simulink model "opv_HDL_Coder_input"  (R2023a)
settings: Solver=VariableStepAuto  StartTime=0.0  StopTime=4*(1/sample_rate)  RelTol=1e-3
values from neighbouring files (symbols this model uses):
  sample_rate = samples_per_symbol*symbol_rate    (= 271000)    [opv.m]
libraries: hdlsllib x2, dspsigops x1
settings Model: Creator=matt  LastModifiedBy=matt

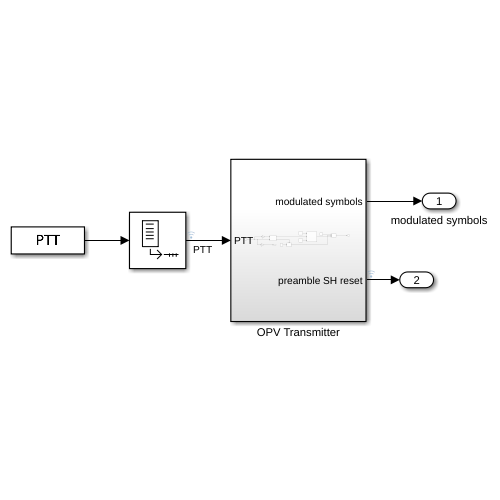
[thumbnail: Simulink's stored preview of the top-level diagram]
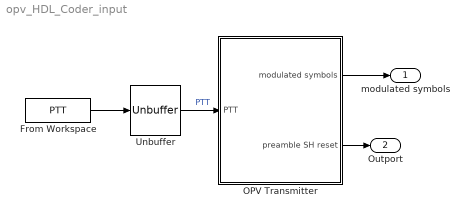
== system opv_HDL_Coder_input ==
  From Workspace : FromWorkspace  VariableName=PTT  OutDataTypeStr=boolean  SampleTime=1/sample_rate
  OPV Transmitter : Subsystem
      settings: LibrarySourceBlock=|
      | hdlsllib/Ports &
      | Subsystems/Subsystem
  Unbuffer : Unbuffer
  modulated symbols : Outport
  Outport : Outport  Port=2
  wires:
  From Workspace/1 -> Unbuffer/1
  Unbuffer/1 -> OPV Transmitter/1(PTT)  "PTT"
  OPV Transmitter/1(modulated symbols) -> modulated symbols/1
  OPV Transmitter/2(preamble SH reset) -> Outport/1

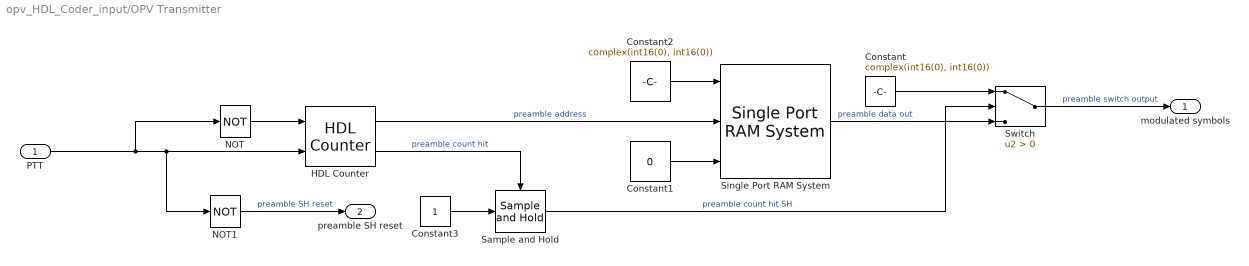
== system opv_HDL_Coder_input/OPV Transmitter ==
  PTT : Inport
  Constant : Constant  Value=complex(int16(0), int16(0))
  Constant1 : Constant  Value=0  VectorParams1D=off  OutDataTypeStr=boolean  SampleTime=-1
  Constant2 : Constant  Value=complex(int16(0), int16(0))  VectorParams1D=off  OutMin=[-32768]  OutMax=32767  OutDataTypeStr=fixdt(1,16,0)  SampleTime=-1
  Constant3 : Constant
  HDL Counter : hdlsllib/Sources/HDL Counter  CountType=Count limited  CountInit=0  CountStep=1  CountMax=255  CountFromType=Initial value  CountFrom=0  CountResetPort=on  CountLoadPort=off  CountEnbPort=on  CountDirPort=off  CountHitOutputPort=on  CountDataType=Unsigned  CountWordLen=8  CountFracLen=0  CountSampTime=1
  NOT : Logic  Operator=NOT  IconShape=distinctive  AllPortsSameDT=off  OutDataTypeStr=boolean
  NOT1 : Logic  Operator=NOT  IconShape=distinctive  AllPortsSameDT=off  OutDataTypeStr=boolean
  Sample and Hold : dspsigops/Sample and Hold  trig=Rising edge  initCond=0  latchinput=off
  Single Port RAM System : hdlsllib/HDL RAMs/Single Port RAM System  RAMType=Single port  WriteOutputValue=New data  RAMInitialValue=1+1i  SimulateUsing=Code generation
  Switch : Switch  Criteria=u2 > Threshold  SaturateOnIntegerOverflow=off  InputSameDT=off
  modulated symbols : Outport
  preamble SH reset : Outport  Port=2
  wires:
  PTT/1 -> NOT/1, NOT1/1, HDL Counter/2
  NOT/1 -> HDL Counter/1
  HDL Counter/1 -> Single Port RAM System/2  "preamble address"
  Constant/1 -> Switch/1
  HDL Counter/2 -> Sample and Hold/Trigger  "preamble count hit"
  Sample and Hold/1 -> Switch/2  "preamble count hit SH"
  NOT1/1 -> preamble SH reset/1  "preamble SH reset"
  Constant1/1 -> Single Port RAM System/3
  Single Port RAM System/1 -> Switch/3  "preamble data out"
  Constant2/1 -> Single Port RAM System/1
  Switch/1 -> modulated symbols/1  "preamble switch output"
  Constant3/1 -> Sample and Hold/1
